simulink model "bus_outputAsBus"  (Simulink 8.0)
settings: Solver=ode45  StartTime=0.0  StopTime=10.0  RelTol=1e-3
settings Model: Creator=massif  LastModifiedBy=massif

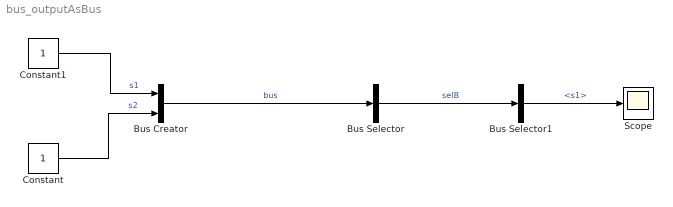
== system bus_outputAsBus ==
  Bus Creator : BusCreator  Inputs=2
  Bus Selector : BusSelector  OutputSignals=s1,s2  OutputAsBus=on
  Bus Selector1 : BusSelector  OutputSignals=s1
  Constant : Constant
  Constant1 : Constant
  Scope : Scope
  wires:
  Constant1/1 -> Bus Creator/1  "s1"
  Bus Creator/1 -> Bus Selector/1  "bus"
  Bus Selector/1 -> Bus Selector1/1  "selB"
  Constant/1 -> Bus Creator/2  "s2"
  Bus Selector1/1 -> Scope/1  "<s1>"
